simulink model "ACAC_DAB_MRAC"  (R2021a)
settings: Solver=VariableStepAuto  StartTime=0.0  StopTime=TSIM  MaxStep=min_step_size  RelTol=1e-3
values from neighbouring files (symbols this model uses):
  am = 1000    [Init_file.m]    (also in Init_file_acac.m = 250; ode_dab_model.m = 581.93)
  ar_0 = 0    [Init_file.m]    (also in Init_file_acac.m; ode_dab_model.m)
  ax_0 = 0    [Init_file.m]    (also in Init_file_acac.m; ode_dab_model.m)
  bm = 1000    [Init_file.m]    (also in Init_file_acac.m = 250; ode_dab_model.m = 581.93)
  f = 10e+3    (= 10000)    [Init_file.m]    (also in Init_file_acac.m = 30000; ode_dab_model.m = -xp/((Rload+Rc)*Co))
  fg = 60    [Init_file_acac.m]
  gamma = 1.5    [Init_file.m]    (also in Init_file_acac.m = 0.5; ode_dab_model.m = 0.04)
  phi_init = 15    [Init_file.m]    (also in Init_file_acac.m)
  voltage_step_time = 0.09    [Init_file.m]    (also in Init_file_acac.m)
  Vout1 = 28    [Init_file.m]    (also in Init_file_acac.m)
  Vout2 = 18    [Init_file.m]    (also in Init_file_acac.m)
undefined symbols (not defined in the file or in its folder): plecs
libraries: dspsrcs4 x1, simulink x1
settings Model: Creator=kvkhh  LastModifiedBy=kvkhh
settings SolverCC: MaxConsecutiveZCs=1000000  ZeroCrossAlgorithm=Adaptive
settings DataIOCC: ReturnWorkspaceOutputs=off
settings DebuggingCC: MaxConsecutiveZCsMsg=none

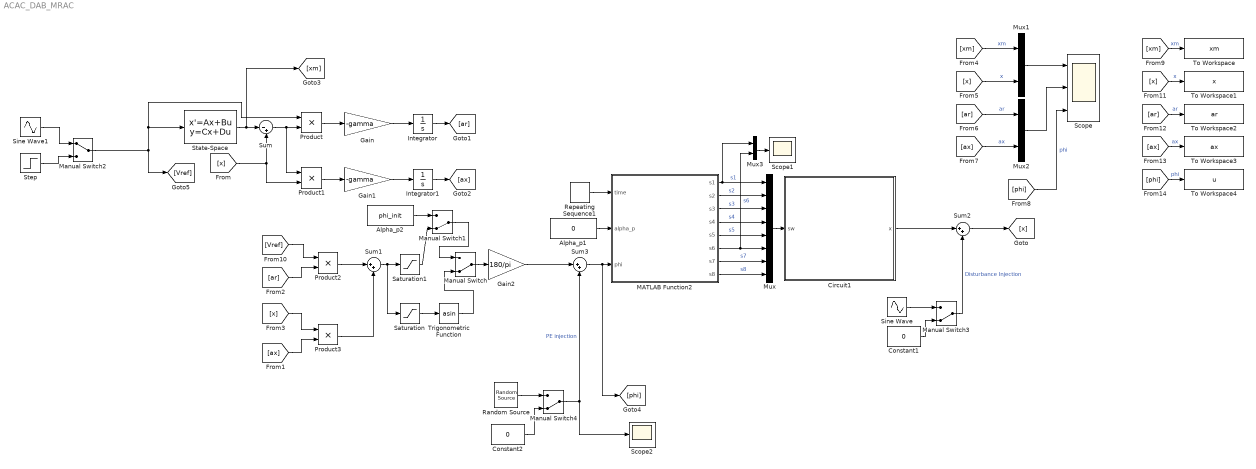
== system ACAC_DAB_MRAC ==
  Alpha_p1 : Constant  Value=0
  Alpha_p2 : Constant  Value=phi_init
  Circuit1 : Subsystem  LoadFcn=plecs('sl', 200);  InitFcn=plecs('sl', 214);  StartFcn=plecs('sl', 208);  StopFcn=plecs('sl', 209);  mask(PlecsCircuit){REPLACE_WITH_PLECS_VAR=REPLACE_WITH_PLECSCIRCUIT_CODE, PLECSData=<binary blob, 4432 chars, not shown>}
      mask prompts: REPLACE_WITH_PLECS_VAR "PLECS Data (Do not delete or modify!)"; PLECSData "PLECS Data (Do not delete or modify!)"
      mask init:
      | % PLACE CUSTOM INITIALIZATIONS ABOVE
      | % DO NOT REMOVE
      | plecs('sl', 215);
      | % DO NOT REMOVE
      settings: CopyFcn=plecs('sl', 203);  DeleteFcn=plecs('sl', 205);  UndoDeleteFcn=plecs('sl', 206);  PreSaveFcn=plecs('sl', 211);  PostSaveFcn=plecs('sl', 201);  NameChangeFcn=plecs('sl', 210);  DestroyFcn=plecs('sl', 207);  PreCopyFcn=plecs('sl', 216);  OpenFcn=plecs('sl', 202);  ErrorFcn=plerrorfcn
      mask Help: web(['file:///' fullfile(plecsdoc, 'creatingacircuit.html')])
      mask Display: disp('PLECS\nCircuit')
  Constant1 : Constant  Value=0
  Constant2 : Constant  Value=0
  Gain : Gain  Gain=-gamma
  Gain1 : Gain  Gain=-gamma
  Gain2 : Gain  Gain=180/pi
  Integrator : Integrator  InitialCondition=ar_0
  Integrator1 : Integrator  InitialCondition=ax_0
  MATLAB Function2 : MATLAB Function  TreatAsAtomicUnit=on
  Manual Switch{,1,3..4} (4 alike) : ManualSwitch  CurrentSetting=0
  Manual Switch2 : ManualSwitch
  Mux : Mux  Inputs=8
  Mux1 : Mux  Inputs=2
  Mux2 : Mux  Inputs=2
  Mux3 : Mux  Inputs=2
  Product{,1..3} (4 alike) : Product
  Random Source : dspsrcs4/Random Source  SrcType=Uniform  NormMethod=Ziggurat  CltLength=12  MinVal=-25  MaxVal=25  MeanVal=0  VarVal=1  RepMode=Not repeatable  rawSeed=1  IsInherit=off  SampMode=Continuous  SampTime=1  SampFrame=1  DataType=Double  OutComplex=Real  OutputFrames=off
  Repeating Sequence1 : simulink/Sources/Repeating Sequence  rep_seq_t=[0 1/f]  rep_seq_y=[0 1]
  Saturation : Saturate  UpperLimit=1  LowerLimit=-1
  Saturation1 : Saturate  UpperLimit=pi/2  LowerLimit=-pi/2
  Scope : Scope  NumInputPorts=3
  Scope1 : Scope
  Scope2 : Scope
  Sine Wave : Sin  Amplitude=2.5  Frequency=100e+3  SampleTime=0
  Sine Wave1 : Sin  Amplitude=Vout1  Frequency=2*pi*fg  SampleTime=0
  State-Space : StateSpace  A=-am  B=bm  D=0  InitialCondition=0
  Step : Step  Time=voltage_step_time  Before=Vout1  After=Vout2  SampleTime=0
  Sum : Sum  Inputs=|-+
  Sum1 : Sum  Inputs=|++
  Sum2 : Sum  Inputs=|++
  Sum3 : Sum  Inputs=|++
  To Workspace : ToWorkspace  VariableName=xm  SaveFormat=Structure With Time  SampleTime=-1
  To Workspace1 : ToWorkspace  VariableName=x  SaveFormat=Structure With Time  SampleTime=-1
  To Workspace2 : ToWorkspace  VariableName=ar  SaveFormat=Structure With Time  SampleTime=-1
  To Workspace3 : ToWorkspace  VariableName=ax  SaveFormat=Structure With Time  SampleTime=-1
  To Workspace4 : ToWorkspace  VariableName=u  SaveFormat=Structure With Time  SampleTime=-1
  Trigonometric Function : Trigonometry  Operator=asin
  wires:
  State-Space/1 -> [xm], Sum/1
  [x] -> Product1/2, Sum/2
  Sum/1 -> Product1/1, Product/2
  Product/1 -> Gain/1
  Product1/1 -> Gain1/1
  Gain/1 -> Integrator/1
  Gain1/1 -> Integrator1/1
  Integrator/1 -> [ar]
  Integrator1/1 -> [ax]
  [ar] -> Product2/2
  [Vref] -> Product2/1
  [x] -> Product3/1
  [ax] -> Product3/2
  Product2/1 -> Sum1/1
  Product3/1 -> Sum1/2
  Sum1/1 -> Saturation/1, Saturation1/1
  Saturation/1 -> Trigonometric Function/1
  Alpha_p1/1 -> MATLAB Function2/2(alpha_p)
  Repeating Sequence1/1 -> MATLAB Function2/1(time)
  MATLAB Function2/1(s1) -> Mux3/1, Mux/1  "s1"
  MATLAB Function2/2(s2) -> Mux/2  "s2"
  MATLAB Function2/3(s3) -> Mux/3  "s3"
  MATLAB Function2/4(s4) -> Mux/4  "s4"
  MATLAB Function2/5(s5) -> Mux/5  "s5"
  MATLAB Function2/6(s6) -> Mux3/2, Mux/6  "s6"
  MATLAB Function2/7(s7) -> Mux/7  "s7"
  MATLAB Function2/8(s8) -> Mux/8  "s8"
  Mux/1 -> Circuit1/1(sw)
  [xm] -> Mux1/1  "xm"
  [x] -> Mux1/2  "x"
  Mux1/1 -> Scope/1
  [ar] -> Mux2/1  "ar"
  [ax] -> Mux2/2  "ax"
  Mux2/1 -> Scope/2
  [phi] -> Scope/3  "phi"
  Trigonometric Function/1 -> Manual Switch/2
  Alpha_p2/1 -> Manual Switch1/1
  Saturation1/1 -> Manual Switch1/2
  Manual Switch1/1 -> Manual Switch/1
  Manual Switch/1 -> Gain2/1
  Mux3/1 -> Scope1/1
  Sine Wave1/1 -> Manual Switch2/1
  Step/1 -> Manual Switch2/2
  Constant1/1 -> Manual Switch3/2
  Sine Wave/1 -> Manual Switch3/1
  Manual Switch3/1 -> Sum2/2  "Disturbance Injection"
  Circuit1/1(x) -> Sum2/1
  Sum2/1 -> [x]
  Manual Switch2/1 -> State-Space/1, Product/1, [Vref]
  Gain2/1 -> Sum3/1
  Sum3/1 -> [phi], MATLAB Function2/3(phi)
  Random Source/1 -> Manual Switch4/1
  Manual Switch4/1 -> Sum3/2, Scope2/1  "PE injection"
  Constant2/1 -> Manual Switch4/2
  [xm] -> To Workspace/1  "xm"
  [x] -> To Workspace1/1  "x"
  [ar] -> To Workspace2/1  "ar"
  [ax] -> To Workspace3/1  "ax"
  [phi] -> To Workspace4/1  "phi"

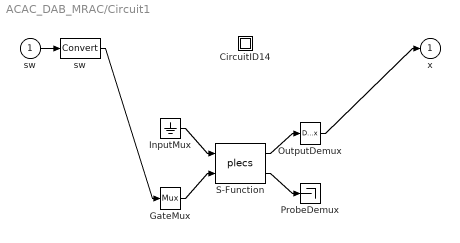
== system ACAC_DAB_MRAC/Circuit1 ==
  sw : Inport  PortDimensions=8
  " CircuitID14 " : Subsystem
  " GateMux " : Mux  Inputs=[ 8 ]
  " InputMux " : Ground
  " OutputDemux " : Demux  Outputs=[ 1 ]
  " ProbeDemux " : Terminator
  " S-Function " : S-Function  FunctionName=plecs  SFunctionDeploymentMode=off  EnableBusSupport=off
  " sw " : DataTypeConversion  SaturateOnIntegerOverflow=on  RndMeth=Zero
  x : Outport  PortDimensions=1
  wires:
  " InputMux "/1 -> " S-Function "/1
  " GateMux "/1 -> " S-Function "/2
  " S-Function "/1 -> " OutputDemux "/1
  " S-Function "/2 -> " ProbeDemux "/1
  sw/1 -> " sw "/1
  " sw "/1 -> " GateMux "/1
  " OutputDemux "/1 -> x/1

== system ACAC_DAB_MRAC/Circuit1/ CircuitID14  ==

== matlab function ACAC_DAB_MRAC/MATLAB Function2 ==
  data: time input; s1 output; alpha_p input; s2 output; s3 output; s4 output; phi input; s5 output; s6 output; s7 output; s8 output
function [s1, s2, s3, s4, s5, s6, s7, s8]  = primary_PWM(time, alpha_p, phi)
%T = 1/fsw;
max_val = 1;

alpha_pr = alpha_p * pi/180; %converting to radians
phi_r = abs(phi) * pi/180;

p1 = max_val*(pi-alpha_pr)/(2*pi);
p2 = max_val*(alpha_pr)/(2*pi);

p3 = max_val*(phi_r)/(2*pi);
p4 = max_val*(pi)/(2*pi);
p5 = max_val*(pi - phi_r)/(2*pi);

%primary side switching
if time <= p1
    s1 = 1;
    s2 = 0;
    s3 = 0;
    s4 = 1;
    
elseif time <= p1 + p2
    s1 = 0;
    s2 = 1;
    s3 = 0;
    s4 = 1;
    
elseif time <= p1 + p2 + p1
    s1 = 0;
    s2 = 1;
    s3 = 1;
    s4 = 0;
    
elseif time <= p1 + p2 + p1 + p2
    s1 = 0;
    s2 = 1;
    s3 = 0;
    s4 = 1;
else
    s1 = 0;
    s2 = 0;
    s3 = 0;
    s4 = 0;
end


%secondary side switching
if phi >= 0
    if time <= p3
        s5 = 0;
        s6 = 1;
        s7 = 1;
        s8 = 0;
        
    elseif time <= p3 + p4
        s5 = 1;
        s6 = 0;
        s7 = 0;
        s8 = 1;
        
    elseif time <= p3 + p4 + p5
        s5 = 0;
        s6 = 1;
        s7 = 1;
        s8 = 0;
    else
        s5 = 0;
        s6 = 0;
        s7 = 0;
        s8 = 0;
    end
elseif phi < 0
    if time <= p5
        s5 = 1;
        s6 = 0;
        s7 = 0;
        s8 = 1;
        
    elseif time <= p4 + p5
        s5 = 0;
        s6 = 1;
        s7 = 1;
        s8 = 0;
        
    elseif time <= p3 + p4 + p5
        s5 = 1;
        s6 = 0;
        s7 = 0;
        s8 = 1;
    else
        s5 = 0;
        s6 = 0;
        s7 = 0;
        s8 = 0;
    end
else
    s5 = 0;
    s6 = 0;
    s7 = 0;
    s8 = 0;
end
